simulink model "Problem__1"  (R2022b)
settings: Solver=VariableStepAuto  StartTime=0.0  StopTime=1000  MaxStep=0.01  RelTol=1e-3
libraries: slpidlib x5, simulink x4
settings Model: Creator=honza  LastModifiedBy=honza
settings OptimizationCC: BlockReduction=off  DefaultParameterBehavior=Inlined  BufferReuse=off

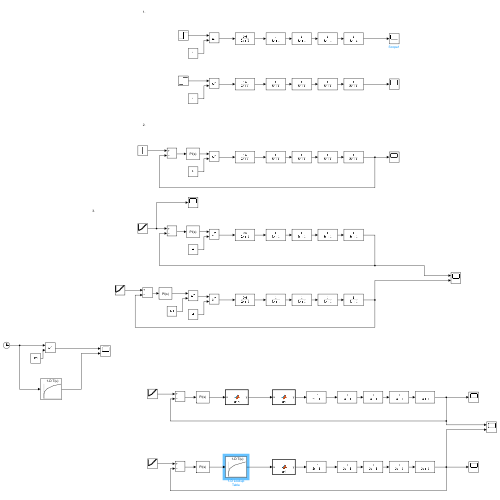
[thumbnail: Simulink's stored preview of the top-level diagram]
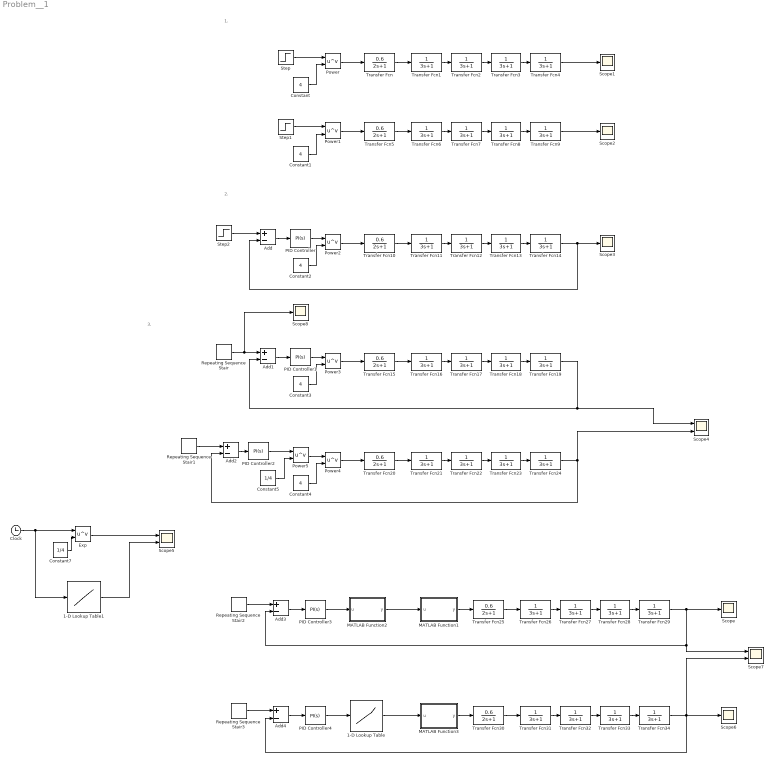
== system Problem__1 ==
  note: 3.
  note: 2.
  note: 1.
  1-D Lookup Table : Lookup_n-D  NumberOfTableDimensions=1  BreakpointsForDimension1=[0 0.01 0.05 0.2 0.57]  Table=[0 0.316 0.473 0.669 0.869]  InternalRulePriority=Speed  RndMeth=Simplest
  1-D Lookup Table1 : Lookup_n-D  NumberOfTableDimensions=1  BreakpointsForDimension1=[0 0.01 0.05 0.2 0.57 1]  Table=[0 0.316 0.473 0.669 0.869 1]  InternalRulePriority=Speed  RndMeth=Simplest
  Add{,1..4} (5 alike) : Sum  Inputs=+-
  Clock : Clock
  Constant{,1..4} (5 alike) : Constant  Value=4
  Constant5 : Constant  Value=1/4
  Constant7 : Constant  Value=1/4
  Exp : Math  Operator=pow
  MATLAB Function1 : MATLAB Function  TreatAsAtomicUnit=on
  MATLAB Function2 : MATLAB Function  TreatAsAtomicUnit=on
  MATLAB Function3 : MATLAB Function  TreatAsAtomicUnit=on
  PID Controller{,1..4} (5 alike) : slpidlib/PID Controller  Controller=PI  Form=Ideal  TimeDomain=Continuous-time  UseExternalTs=off  SampleTime=-1  IntegratorMethod=Forward Euler  FilterMethod=Forward Euler  ControllerParametersSource=internal  P=10/(0.6*12.2)  I=1/10  UseKiTs=off  D=0  N=100  UseFilter=on  TunerSelectOption=Transfer Function Based (PID Tuner App)  InitialConditionSource=internal  InitialConditionForIntegrator=0  InitialConditionForFilter=0  DifferentiatorICPrevScaledInput=0  ExternalReset=none  TrackingMode=off  Kt=1  LimitOutput=off  SatLimitsSource=internal  UpperSaturationLimit=inf  LowerSaturationLimit=-inf  LinearizeAsGain=on  AntiWindupMode=none  Kb=1  LimitIntegrator=off  UpperIntegratorSaturationLimit=inf  LowerIntegratorSaturationLimit=-inf  POutMin=[]  POutMax=[]  IOutMin=[]  IOutMax=[]  DOutMin=[]  DOutMax=[]  NOutMin=[]  NOutMax=[]  SumOutMin=[]  SumOutMax=[]  SaturationOutMin=[]  SaturationOutMax=[]  PParamMin=[]  PParamMax=[]  IParamMin=[]  IParamMax=[]  DParamMin=[]  DParamMax=[]  NParamMin=[]  NParamMax=[]  KbParamMin=[]  KbParamMax=[]  KtParamMin=[]  KtParamMax=[]  KbOutMin=[]  KbOutMax=[]  KtOutMin=[]  KtOutMax=[]  IntegratorOutMin=[]  IntegratorOutMax=[]  FilterOutMin=[]  FilterOutMax=[]  SumI1OutMin=[]  SumI1OutMax=[]  SumI2OutMin=[]  SumI2OutMax=[]  SumI3OutMin=[]  SumI3OutMax=[]  SumI4OutMin=[]  SumI4OutMax=[]  SumDOutMin=[]  SumDOutMax=[]  DifferentiatorOutMin=[]  DifferentiatorOutMax=[]  FilterDiffOutCoefMin=[]  FilterDiffOutCoefMax=[]  ReciprocalOutMin=[]  ReciprocalOutMax=[]  SumDenOutMin=[]  SumDenOutMax=[]  SumNumOutMin=[]  SumNumOutMax=[]  DivideOutMin=[]  DivideOutMax=[]  UdiffTsProdOutMin=[]  UdiffTsProdOutMax=[]  NTsProdOutMin=[]  NTsProdOutMax=[]  UintegralTsProdOutMin=[]  UintegralTsProdOutMax=[]  UngainTsProdOutMin=[]  UngainTsProdOutMax=[]  ClampingZeroOutDataTypeStr=Inherit: Inherit via back propagation  ClampingZeroOutMin=[]  ClampingZeroOutMax=[]  FilterDenConstantOutDataTypeStr=Inherit: Inherit via back propagation  FilterDenConstantOutMin=[]  FilterDenConstantOutMax=[]  PCopyOutDataTypeStr=Inherit: Inherit via back propagation  PCopyOutMin=[]  PCopyOutMax=[]  NCopyOutDataTypeStr=Inherit: Inherit via back propagation  NCopyOutMin=[]  NCopyOutMax=[]  IntegratorContinuousStateAttributes=''  IntegratorStateMustResolveToSignalObject=off  IntegratorRTWStateStorageClass=Auto  FilterContinuousStateAttributes=''  FilterStateMustResolveToSignalObject=off  FilterRTWStateStorageClass=Auto  ParallelPVariant=Passthrough  IdealPVariant=InternalParameters  IVariant=InternalParameters  DVariant=Disabled  IntegratorVariant=Continuous  SatVariant=Disabled  AWVariant=Passthrough  PCopyVariant=Disabled  TRVariant=Disabled  FdbkBlocksVariant=Forward  IdealPFdbkVariant=Disabled  SatFdbkVariant=Disabled  DerivativeFilterVariant=Disabled  NVariant=Disabled  NCopyVariant=Disabled_SignalSpec  FilterICVariant=Disabled  IntegratorICVariant=InternalICs  ExternalResetVariant=Disabled  TRSumVariant=Passthrough  SumFdbkVariant=Disabled  SumVariant=Sum_PI  TsampFilterVariant=InternalTs  TsampNgainVariant=Passthrough  TsampIntegralVariant=Passthrough  ExternalSaturationOutDataTypeStr=Inherit: Same as second input
  Power{,1..5} (6 alike) : Math  Operator=pow
  Repeating Sequence Stair : simulink/Sources/Repeating Sequence Stair  OutValues=[0.01 0.05 0.1 0.2 0.3 0.4 0.5].'  tsamp=300  OutMin=[]  OutMax=[]  OutDataTypeStr=double  OutputDataTypeScalingMode=double  OutDataType=fixdt(0,8)  ConRadixGroup=Best Precision: Vector-wise  OutScaling=2^-12
  Repeating Sequence Stair1 : simulink/Sources/Repeating Sequence Stair  OutValues=[0.01 0.05 0.1 0.2 0.3 0.4 0.5].'  tsamp=300  OutMin=[]  OutMax=[]  OutDataTypeStr=double  OutputDataTypeScalingMode=double  OutDataType=fixdt(0,8)  ConRadixGroup=Best Precision: Vector-wise  OutScaling=2^-12
  Repeating Sequence Stair2 : simulink/Sources/Repeating Sequence Stair  OutValues=[0.01 0.05 0.1 0.2 0.3 0.4 0.5].'  tsamp=200  OutMin=[]  OutMax=[]  OutDataTypeStr=double  OutputDataTypeScalingMode=double  OutDataType=fixdt(0,8)  ConRadixGroup=Best Precision: Vector-wise  OutScaling=2^-12
  Repeating Sequence Stair3 : simulink/Sources/Repeating Sequence Stair  OutValues=[0.01 0.05 0.1 0.2 0.3 0.4 0.5].'  tsamp=200  OutMin=[]  OutMax=[]  OutDataTypeStr=double  OutputDataTypeScalingMode=double  OutDataType=fixdt(0,8)  ConRadixGroup=Best Precision: Vector-wise  OutScaling=2^-12
  Scope{,1..3,6,8} (6 alike) : Scope
  Scope4 : Scope  NumInputPorts=2
  Scope5 : Scope  NumInputPorts=2
  Scope7 : Scope  NumInputPorts=2
  Step : Step  Time=0  After=0.05  SampleTime=0
  Step1 : Step  Time=50  Before=0.8  After=0.85  SampleTime=0
  Step2 : Step  After=0.05  SampleTime=0
  Transfer Fcn{,5,10,15,20,25,30} (7 alike) : TransferFcn  Numerator=[0.6]  Denominator=[2 1]
  Transfer Fcn{1..4,6..9,11..14,16..19,21..24,26..29,31..34} (28 alike) : TransferFcn  Denominator=[3 1]
  wires:
  Transfer Fcn3/1 -> Transfer Fcn4/1
  Transfer Fcn2/1 -> Transfer Fcn3/1
  Transfer Fcn1/1 -> Transfer Fcn2/1
  Transfer Fcn/1 -> Transfer Fcn1/1
  Transfer Fcn6/1 -> Transfer Fcn7/1
  Transfer Fcn8/1 -> Transfer Fcn9/1
  Transfer Fcn9/1 -> Scope2/1
  Transfer Fcn7/1 -> Transfer Fcn8/1
  Transfer Fcn5/1 -> Transfer Fcn6/1
  Transfer Fcn4/1 -> Scope1/1
  Power/1 -> Transfer Fcn/1
  Step/1 -> Power/1
  Constant/1 -> Power/2
  Power1/1 -> Transfer Fcn5/1
  Constant1/1 -> Power1/2
  Step1/1 -> Power1/1
  Transfer Fcn14/1 -> Add/2, Scope3/1
  Power2/1 -> Transfer Fcn10/1
  Transfer Fcn11/1 -> Transfer Fcn12/1
  Transfer Fcn13/1 -> Transfer Fcn14/1
  Transfer Fcn12/1 -> Transfer Fcn13/1
  Constant2/1 -> Power2/2
  Transfer Fcn10/1 -> Transfer Fcn11/1
  PID Controller/1 -> Power2/1
  Step2/1 -> Add/1
  Add/1 -> PID Controller/1
  Add1/1 -> PID Controller1/1
  Repeating Sequence Stair/1 -> Scope8/1, Add1/1
  Transfer Fcn17/1 -> Transfer Fcn18/1
  Transfer Fcn18/1 -> Transfer Fcn19/1
  PID Controller1/1 -> Power3/1
  Constant3/1 -> Power3/2
  Transfer Fcn15/1 -> Transfer Fcn16/1
  Transfer Fcn19/1 -> Add1/2, Scope4/1
  Transfer Fcn16/1 -> Transfer Fcn17/1
  Power3/1 -> Transfer Fcn15/1
  Repeating Sequence Stair1/1 -> Add2/1
  Power4/1 -> Transfer Fcn20/1
  Transfer Fcn20/1 -> Transfer Fcn21/1
  Transfer Fcn22/1 -> Transfer Fcn23/1
  Transfer Fcn23/1 -> Transfer Fcn24/1
  Constant4/1 -> Power4/2
  Transfer Fcn21/1 -> Transfer Fcn22/1
  Add2/1 -> PID Controller2/1
  Transfer Fcn24/1 -> Scope4/2, Add2/2
  Constant5/1 -> Power5/2
  Power5/1 -> Power4/1
  PID Controller2/1 -> Power5/1
  Transfer Fcn29/1 -> Scope/1, Scope7/1, Add3/2
  Add3/1 -> PID Controller3/1
  Transfer Fcn28/1 -> Transfer Fcn29/1
  Repeating Sequence Stair2/1 -> Add3/1
  Transfer Fcn27/1 -> Transfer Fcn28/1
  Transfer Fcn25/1 -> Transfer Fcn26/1
  Transfer Fcn26/1 -> Transfer Fcn27/1
  MATLAB Function1/1(y) -> Transfer Fcn25/1
  MATLAB Function2/1(y) -> MATLAB Function1/1(u)
  PID Controller3/1 -> MATLAB Function2/1(u)
  Clock/1 -> 1-D Lookup Table1/1, Exp/1
  Constant7/1 -> Exp/2
  Exp/1 -> Scope5/1
  PID Controller4/1 -> 1-D Lookup Table/1
  Transfer Fcn31/1 -> Transfer Fcn32/1
  Transfer Fcn30/1 -> Transfer Fcn31/1
  Repeating Sequence Stair3/1 -> Add4/1
  Add4/1 -> PID Controller4/1
  Transfer Fcn33/1 -> Transfer Fcn34/1
  Transfer Fcn34/1 -> Add4/2, Scope7/2, Scope6/1
  1-D Lookup Table/1 -> MATLAB Function3/1(u)
  Transfer Fcn32/1 -> Transfer Fcn33/1
  MATLAB Function3/1(y) -> Transfer Fcn30/1
  1-D Lookup Table1/1 -> Scope5/2

== matlab function Problem__1/MATLAB Function2 ==
  data: u input; y output
function y = u14(u)

y = u^(1/4);




% 0.bod (0, 0)
% 1.bod (0.05, 0.47)
% 2.bod (0.32, 0.75)
% 3.bod (1, 1)
%
% směrnice
% 1. primka (0.47)
% 2. primka (0.39)
% 3. primka (0.72)

== matlab function Problem__1/MATLAB Function3 ==
  data: u input; y output
function y = u4(u)

y = u^4;

== matlab function Problem__1/MATLAB Function1 ==
  data: u input; y output
function y = u4(u)

y = u^4;
